simulink model "cps_physics_linearize_harness_v2"  (R2012b)
settings: Solver=ode14x  SolverMode=SingleTasking  StartTime=0.0  StopTime=6  FixedStep=0.005  RelTol=1e-2
model workspace (MAT data in the model file):
  ini_G_block_hpos = -0.4
  ini_G_block_vpos = 0.14
  block_height = 0.07
  ini_nozzle_pos = 0.3
  board_vpos = 0
  blockG = 1
  blockR = 2
  ini_R_block_vpos = 0.07
  ini_R_block_hpos = -0.4
  ini_B_block_vpos = 0.21
  ini_B_block_hpos = -0.4
libraries: fl_lib x6, nesl_utility x3, simulink x1
settings Model: Creator=pmosterm  LastModifiedBy=pmosterm
settings SolverCC: EnableConcurrentExecution=on  ConcurrentTasks=on
settings DataIOCC: SignalLoggingSaveFormat=ModelDataLogs

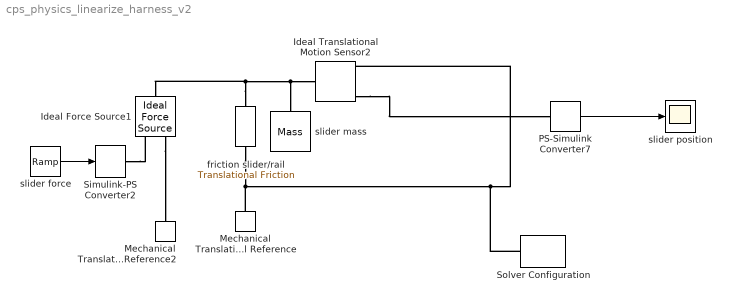
== system cps_physics_linearize_harness_v2 ==
  Ideal Force Source1 : fl_lib/Mechanical/Mechanical Sources/Ideal Force Source  v_Log=off  f_Log=off  LocalVarNames=|v|f  LocalVarDescs=|v|f  LocalVarLogging=[0 0]
  Ideal Translational Motion Sensor2 : fl_lib/Mechanical/Mechanical Sensors/Ideal Translational Motion Sensor  offset=0 m  v_Log=off  f_Log=off  x_Log=off  LocalVarNames=|v|f|x  LocalVarDescs=|v|f|x  LocalVarLogging=[0 0 0]
  Mechanical Translational Reference : fl_lib/Mechanical/Translational Elements/Mechanical Translational Reference  f_Log=off  LocalVarNames=|f  LocalVarDescs=|f  LocalVarLogging=0
  Mechanical Translational Reference2 : fl_lib/Mechanical/Translational Elements/Mechanical Translational Reference  f_Log=off  LocalVarNames=|f  LocalVarDescs=|f  LocalVarLogging=0
  PS-Simulink Converter7 : nesl_utility/PS-Simulink Converter  PhysicalDomain=network_engine_domain  LeftPortType=input  RightPortType=output  SubClassName=ps_output  PseudoPeriodic=off  Frequencies=[]  Unit=1  AffineConversion=off
  Simulink-PS Converter2 : nesl_utility/Simulink-PS Converter  PhysicalDomain=network_engine_domain  LeftPortType=input  RightPortType=output  SubClassName=ps_input  PseudoPeriodic=off  Frequencies=[]  NoiseDistribution=none  NoiseParameters=[]  Unit=1  AffineConversion=off  InputFilterTimeConstant=.001  UdotUserProvided=0  SimscapeFilterOrder=1  InputFiltering=off
  Solver Configuration : nesl_utility/Solver Configuration  PhysicalDomain=network_engine_domain  LeftPortType=input  RightPortType=generic  SubClassName=solver  Accelerate=off  Profile=off  UseLocalSampling=off  FrequencyDomain=off  Tones=[]  Harmonics=[]  UseCCode=off  SimulateNoise=off  EnableSwitchedLinearOptims=on  DoDC=off  ResidualTolerance=1e-9  UseLocalSolver=off  LocalSolverChoice=NE_BACKWARD_EULER_ADVANCER  LocalSolverSampleTime=.005  DoFixedCost=off  MaxNonlinIter=3  MaxModeIter=2  LinearAlgebra=Sparse  DelaysMemoryBudget=1024
  friction slider/rail : fl_lib/Mechanical/Translational Elements/Translational Friction  brkwy_frc=2.5 N  Col_frc=2 N  visc_coef=10 N/(m/s)  trans_coef=1 s/m  vel_thr=1e-5 m/s  f_Log=off  v_Log=off  LocalVarNames=|f|v  LocalVarDescs=|f|v  LocalVarLogging=[0 0]
  slider force : simulink/Sources/Ramp  slope=1  start=0  X0=0
  slider mass : fl_lib/Mechanical/Translational Elements/Mass  mass=1 kg  initial_velocity=0 m/s  f_Log=off  LocalVarNames=|f  LocalVarDescs=|f  LocalVarLogging=0
  slider position : Scope
      settings: TimeRange=10  YMin=0  YMax=3
  wires:
  PS-Simulink Converter7/1 -> slider position/1
  slider force/1 -> Simulink-PS Converter2/1
  connections:
  friction slider/rail/RConn1 -- Mechanical Translational Reference/LConn1 -- Solver Configuration/RConn1 -- Ideal Translational Motion Sensor2/RConn1
  friction slider/rail/LConn1 -- Ideal Force Source1/LConn1 -- slider mass/LConn1 -- Ideal Translational Motion Sensor2/LConn1
  Ideal Translational Motion Sensor2/RConn3 -- PS-Simulink Converter7/LConn1
  Simulink-PS Converter2/RConn1 -- Ideal Force Source1/RConn1
  Ideal Force Source1/RConn2 -- Mechanical Translational Reference2/LConn1
